simulink model "attitude_interface"  (R2019b)
settings: Solver=FixedStepAuto  StartTime=0.0  StopTime=Inf  FixedStep=FIXED_STEP_SIZE  RelTol=1e-3
values from neighbouring files (symbols this model uses):
  FIXED_STEP_SIZE = 0.01    [Exx6_2.m]
  GAZEBO_SYNC_DT = 0.01    [Exx6_2.m]
  RAD2DEG = 180/pi    (= 57.2957795131)    [Exx6_2.m]
  THRUST_OFFSET = 15    [Exx6_2.m]
undefined symbols (not defined in the file or in its folder): Header, Pitch, Roll, Thrust, YawRate
libraries: robotlib x5, robotgazebolib x1, simulink x1
settings Model: Creator=ananda  LastModifiedBy=ubuntu
settings OptimizationCC: EnhancedBackFolding=on  PassReuseOutputArgsAs=Individual arguments  ZeroExternalMemoryAtStartup=off  ZeroInternalMemoryAtStartup=off  MaxStackSize=64  OptimizeBlockOrder=speed  DifferentSizesBufferReuse=on  OptimizationCustomize=off  EfficientTunableParamExpr=on
settings DebuggingCC: ParameterTunabilityLossMsg=error
settings HardwareCC: ProdBitPerPointer=32  ProdBitPerSizeT=32  ProdBitPerPtrDiffT=32  ProdLargestAtomicFloat=None  ProdIntDivRoundTo=Undefined  ProdEndianess=Unspecified  ProdWordSize=32  ProdHWDeviceType=Generic->Unspecified (assume 32-bit Generic)  UseEmbeddedCoderFeatures=off
settings SFSimCC: MATLABDynamicMemAlloc=off
settings RTWCC: SystemTargetFile=ert.tlc  HardwareBoard=Robot Operating System (ROS)  TLCOptions="-aInlineSetEventsForThisBaseRateFcn=TLC_FALSE -aSuppressMultiTaskScheduler=TLC_FALSE  -aRateBasedStepFcn=0"  TemplateMakefile=ert_default_tmf  GenerateReport=on  Toolchain=Catkin  IncludeHyperlinkInReport=on  LaunchReport=on  TargetLang=C++  GenerateTraceInfo=on  GenerateTraceReport=on  GenerateTraceReportSl=on  GenerateTraceReportSf=on  GenerateTraceReportEml=on
settings CodeAppCC: ForceParamTrailComments=on  IgnoreCustomStorageClasses=off  OperatorAnnotations=on  SimulinkDataObjDesc=on  SFDataObjDesc=on  InsertBlockDesc=on
settings ERTTargetCC: SupportNonInlinedSFcns=on

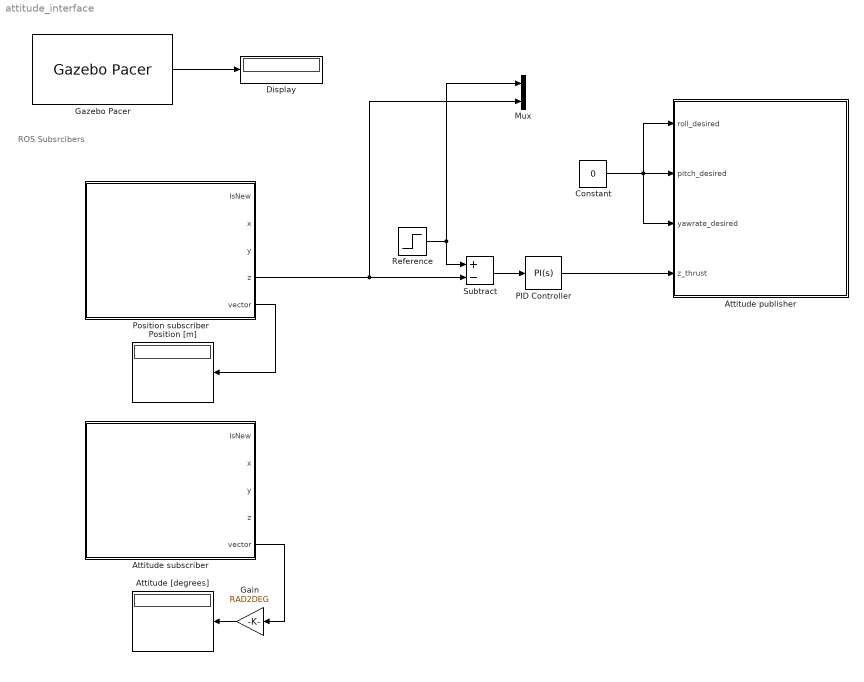
== system attitude_interface ==
  note: ROS Subsrcibers
  Attitude [degrees] : Display
  Attitude publisher : Subsystem
  Attitude subscriber : Subsystem
  Constant : Constant  Value=0
  Display : Display
  Gain : Gain  Gain=RAD2DEG
  Gazebo Pacer : robotgazebolib/Gazebo Pacer  ResetBehavior=Reset Gazebo simulation time  SampleTime=GAZEBO_SYNC_DT
      settings: SourceProductName=Robotics System Toolbox  SourceProductBaseCode=RO
  Mux : Mux  Inputs=2
  PID Controller : simulink/Continuous/PID Controller  Controller=PI  Form=Parallel  TimeDomain=Continuous-time  SampleTime=-1  IntegratorMethod=Forward Euler  FilterMethod=Forward Euler  ControllerParametersSource=internal  P=1  I=1  D=0  UseFilter=on  N=100  TunerSelectOption=Transfer Function Based (PID Tuner App)  InitialConditionSource=internal  InitialConditionForIntegrator=0  InitialConditionForFilter=0  DifferentiatorICPrevScaledInput=0  ExternalReset=none  TrackingMode=off  Kt=1  LimitOutput=off  UpperSaturationLimit=inf  LowerSaturationLimit=-inf  LinearizeAsGain=on  AntiWindupMode=none  Kb=1  POutMin=[]  POutMax=[]  IOutMin=[]  IOutMax=[]  DOutMin=[]  DOutMax=[]  NOutMin=[]  NOutMax=[]  SumOutMin=[]  SumOutMax=[]  SaturationOutMin=[]  SaturationOutMax=[]  PParamMin=[]  PParamMax=[]  IParamMin=[]  IParamMax=[]  DParamMin=[]  DParamMax=[]  NParamMin=[]  NParamMax=[]  KbParamMin=[]  KbParamMax=[]  KtParamMin=[]  KtParamMax=[]  KbOutMin=[]  KbOutMax=[]  KtOutMin=[]  KtOutMax=[]  IntegratorOutMin=[]  IntegratorOutMax=[]  FilterOutMin=[]  FilterOutMax=[]  SumI1OutMin=[]  SumI1OutMax=[]  SumI2OutMin=[]  SumI2OutMax=[]  SumI3OutMin=[]  SumI3OutMax=[]  SumI4OutMin=[]  SumI4OutMax=[]  SumDOutMin=[]  SumDOutMax=[]  DifferentiatorOutMin=[]  DifferentiatorOutMax=[]  FilterDiffOutCoefMin=[]  FilterDiffOutCoefMax=[]  ReciprocalOutMin=[]  ReciprocalOutMax=[]  SumDenOutMin=[]  SumDenOutMax=[]  SumNumOutMin=[]  SumNumOutMax=[]  DivideOutMin=[]  DivideOutMax=[]  IntegratorContinuousStateAttributes=''  IntegratorStateMustResolveToSignalObject=off  IntegratorRTWStateStorageClass=Auto  FilterContinuousStateAttributes=''  FilterStateMustResolveToSignalObject=off  FilterRTWStateStorageClass=Auto  ParallelPVariant=InternalParameters  IdealPVariant=Disabled  IVariant=InternalParameters  DVariant=Disabled  IntegratorVariant=Continuous  SatVariant=Disabled  AWVariant=Passthrough  PCopyVariant=Disabled  TRVariant=Disabled  FdbkBlocksVariant=Forward  IdealPFdbkVariant=Disabled  SatFdbkVariant=Disabled  DerivativeFilterVariant=Disabled  NVariant=Disabled  NCopyVariant=Disabled_SignalSpec  FilterICVariant=Disabled  IntegratorICVariant=InternalICs  ExternalResetVariant=Disabled  TRSumVariant=Passthrough  SumFdbkVariant=Disabled  SumVariant=Sum_PI
  Position [m] : Display
  Position subscriber : Subsystem
  Reference : Step  SampleTime=0
  Subtract : Sum  Inputs=+-
  wires:
  Position subscriber/5(vector) -> Position [m]/1
  Attitude subscriber/5(vector) -> Gain/1
  Gain/1 -> Attitude [degrees]/1
  Gazebo Pacer/1 -> Display/1
  Constant/1 -> Attitude publisher/1(roll_desired), Attitude publisher/3(yawrate_desired), Attitude publisher/2(pitch_desired)
  Position subscriber/4(z) -> Mux/2, Subtract/2
  Reference/1 -> Subtract/1, Mux/1
  Subtract/1 -> PID Controller/1
  PID Controller/1 -> Attitude publisher/4(z_thrust)

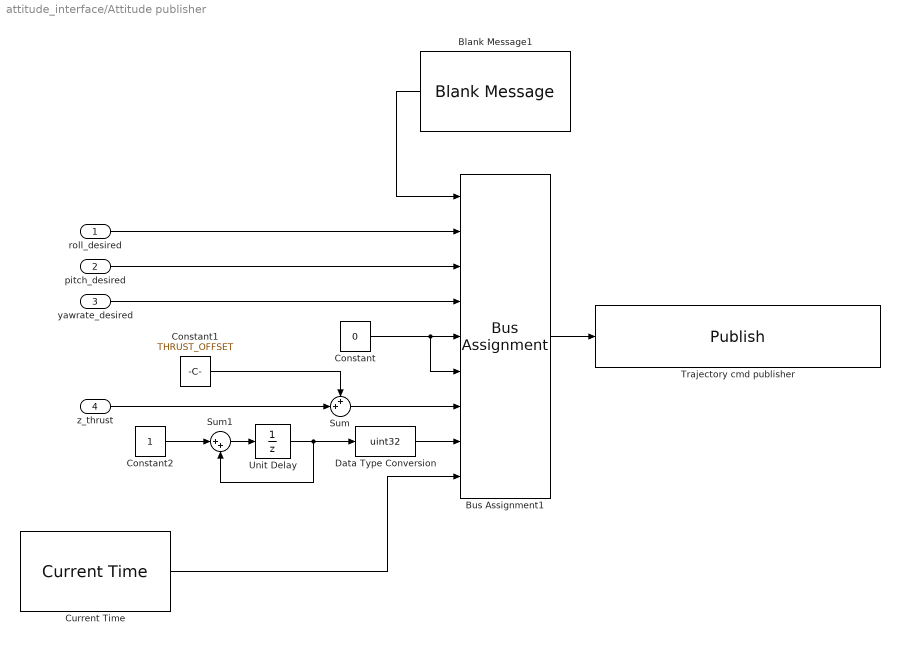
== system attitude_interface/Attitude publisher ==
  roll_desired : Inport
  pitch_desired : Inport  Port=2
  yawrate_desired : Inport  Port=3
  z_thrust : Inport  Port=4
  Blank Message1 : robotlib/Blank Message  messageClass=Message  entityType=mav_msgs/RollPitchYawrateThrust  messageType=mav_msgs/RollPitchYawrateThrust  SampleTime=FIXED_STEP_SIZE
      settings: SourceProductName=ROS Toolbox
  Bus Assignment1 : BusAssignment  AssignedSignals=Roll,Pitch,YawRate,Thrust.X,Thrust.Y,Thrust.Z,Header.Seq,Header.Stamp
  Constant : Constant  Value=0
  Constant1 : Constant  Value=THRUST_OFFSET
  Constant2 : Constant
  Current Time : robotlib/Current Time  OutputFormat=bus  SampleTime=FIXED_STEP_SIZE  ModelName=attitude_interface
      settings: SourceProductName=ROS Toolbox  SourceProductBaseCode=RR
  Data Type Conversion : DataTypeConversion  OutDataTypeStr=uint32
  Sum : Sum  Inputs=++|
  Sum1 : Sum  Inputs=|++
  Trajectory cmd publisher : robotlib/Publish  topicSource=Specify your own  topic=/hummingbird/command/roll_pitch_yawrate_thrust  messageType=mav_msgs/RollPitchYawrateThrust  messageQueueLength=1
      settings: SourceProductName=ROS Toolbox
  Unit Delay : UnitDelay  SampleTime=FIXED_STEP_SIZE  HasFrameUpgradeWarning=on
  wires:
  Bus Assignment1/1 -> Trajectory cmd publisher/1
  Blank Message1/1 -> Bus Assignment1/1
  Constant/1 -> Bus Assignment1/6, Bus Assignment1/5
  yawrate_desired/1 -> Bus Assignment1/4
  pitch_desired/1 -> Bus Assignment1/3
  roll_desired/1 -> Bus Assignment1/2
  Sum/1 -> Bus Assignment1/7
  z_thrust/1 -> Sum/2
  Constant1/1 -> Sum/1
  Sum1/1 -> Unit Delay/1
  Unit Delay/1 -> Sum1/2, Data Type Conversion/1
  Constant2/1 -> Sum1/1
  Current Time/1 -> Bus Assignment1/9
  Data Type Conversion/1 -> Bus Assignment1/8

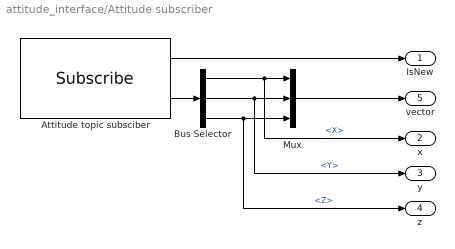
== system attitude_interface/Attitude subscriber ==
  Attitude topic subsciber : robotlib/Subscribe  topicSource=Specify your own  topic=/hummingbird/orientation_rpy  messageType=geometry_msgs/Vector3  sampleTime=ATTI_SUB_DT  messageQueueLength=1
      settings: SourceProductName=ROS Toolbox
  Bus Selector : BusSelector  OutputSignals=X,Y,Z
  Mux : Mux  Inputs=3
  IsNew : Outport
  x : Outport  Port=2
  y : Outport  Port=3
  z : Outport  Port=4
  vector : Outport  Port=5
  wires:
  Bus Selector/3 -> z/1, Mux/3  "<Z>"
  Bus Selector/2 -> y/1, Mux/2  "<Y>"
  Bus Selector/1 -> x/1, Mux/1  "<X>"
  Attitude topic subsciber/2 -> Bus Selector/1
  Attitude topic subsciber/1 -> IsNew/1
  Mux/1 -> vector/1

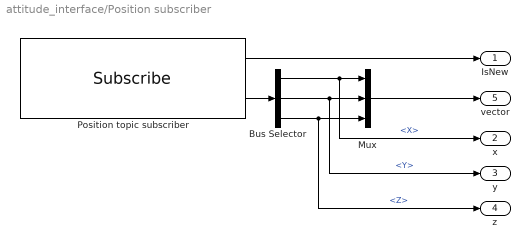
== system attitude_interface/Position subscriber ==
  Bus Selector : BusSelector  OutputSignals=Point.X,Point.Y,Point.Z
  Mux : Mux  Inputs=3
  Position topic subscriber : robotlib/Subscribe  topicSource=Specify your own  topic=/hummingbird/odometry_sensor1/position  messageType=geometry_msgs/PointStamped  sampleTime=POS_SUB_DT  messageQueueLength=1
      settings: SourceProductName=ROS Toolbox
  IsNew : Outport
  x : Outport  Port=2
  y : Outport  Port=3
  z : Outport  Port=4
  vector : Outport  Port=5
  wires:
  Bus Selector/3 -> z/1, Mux/3  "<Z>"
  Bus Selector/2 -> y/1, Mux/2  "<Y>"
  Mux/1 -> vector/1
  Bus Selector/1 -> x/1, Mux/1  "<X>"
  Position topic subscriber/2 -> Bus Selector/1
  Position topic subscriber/1 -> IsNew/1
